simulink model "TST_FanSpd_DD"  (R2016b)
settings: Solver=FixedStepDiscrete  StartTime=0.0  StopTime=simTime  FixedStep=sampleTime  RelTol=1e-3
values from neighbouring files (symbols this model uses):
  testCase = 1    [initTST_FanSpd_DD_001.m]    (also in initTST_FanSpd_DD_002.m = 2)
libraries: simulink x7, UnitTest_Lib x4
settings Model: Creator=xinchangran  LastModifiedBy=xinchangran
settings DebuggingCC: SignalRangeChecking=error

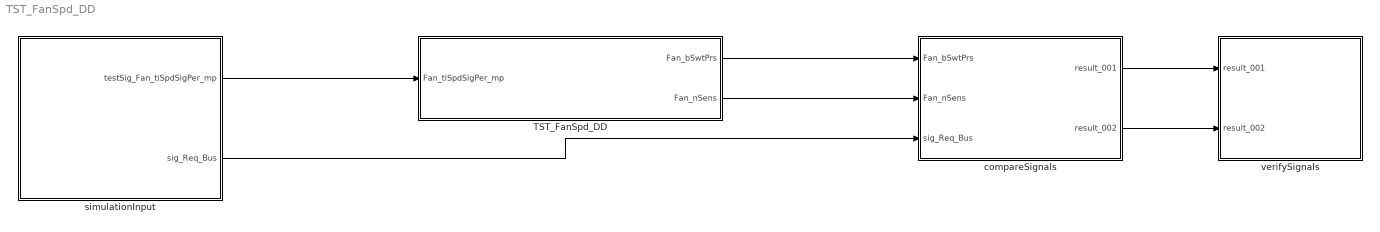
== system TST_FanSpd_DD ==
  TST_FanSpd_DD : Subsystem
  compareSignals : Subsystem
  simulationInput : Subsystem
  verifySignals : Subsystem
  wires:
  simulationInput/1(testSig_Fan_tiSpdSigPer_mp) -> TST_FanSpd_DD/1(Fan_tiSpdSigPer_mp)
  TST_FanSpd_DD/1(Fan_bSwtPrs) -> compareSignals/1(Fan_bSwtPrs)
  TST_FanSpd_DD/2(Fan_nSens) -> compareSignals/2(Fan_nSens)
  simulationInput/2(sig_Req_Bus) -> compareSignals/3(sig_Req_Bus)
  compareSignals/1(result_001) -> verifySignals/1(result_001)
  compareSignals/2(result_002) -> verifySignals/2(result_002)

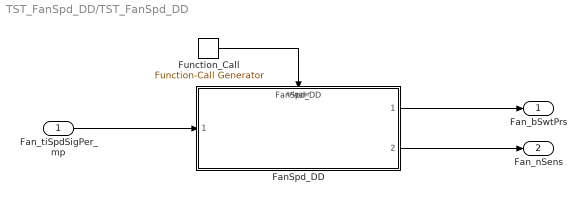
== system TST_FanSpd_DD/TST_FanSpd_DD ==
  Fan_tiSpdSigPer_mp : Inport
  FanSpd_DD : ModelReference  ModelNameDialog=FanSpd_DD  SimulationMode=Normal  ModelReferenceVersion=1.45  TriggerPortName=function  TriggerPortTriggerType=function-call  TriggerPortStatesWhenEnabling=held
  Function_Call : simulink/Ports & Subsystems/Function-Call Generator  sample_time=sampleTime  numberOfIterations=1
  Fan_bSwtPrs : Outport
  Fan_nSens : Outport  Port=2
  wires:
  Function_Call/1 -> FanSpd_DD/Trigger
  Fan_tiSpdSigPer_mp/1 -> FanSpd_DD/1
  FanSpd_DD/1 -> Fan_bSwtPrs/1
  FanSpd_DD/2 -> Fan_nSens/1

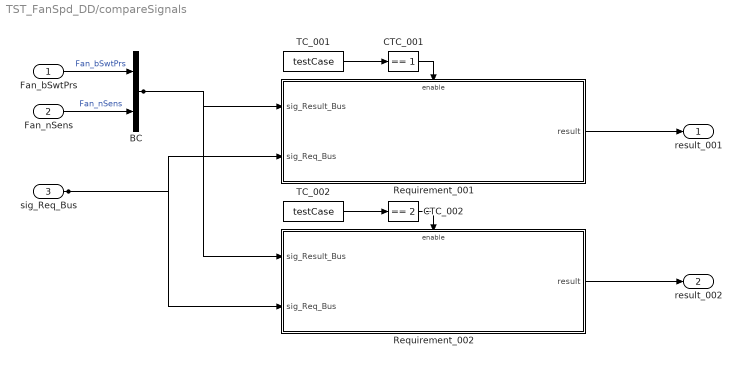
== system TST_FanSpd_DD/compareSignals ==
  Fan_bSwtPrs : Inport
  Fan_nSens : Inport  Port=2
  sig_Req_Bus : Inport  Port=3
  BC : BusCreator  Inputs=2
  CTC_001 : simulink/Logic and Bit Operations/Compare To Constant  relop===  const=1  OutDataTypeStr=boolean
  CTC_002 : simulink/Logic and Bit Operations/Compare To Constant  relop===  const=2  OutDataTypeStr=boolean
  Requirement_001 : Subsystem
  Requirement_002 : Subsystem
  TC_001 : Constant  Value=testCase
  TC_002 : Constant  Value=testCase
  result_001 : Outport
  result_002 : Outport  Port=2
  wires:
  Fan_bSwtPrs/1 -> BC/1  "Fan_bSwtPrs"
  Fan_nSens/1 -> BC/2  "Fan_nSens"
  TC_001/1 -> CTC_001/1
  CTC_001/1 -> Requirement_001/Enable
  sig_Req_Bus/1 -> Requirement_001/2(sig_Req_Bus), Requirement_002/2(sig_Req_Bus)
  BC/1 -> Requirement_001/1(sig_Result_Bus), Requirement_002/1(sig_Result_Bus)
  Requirement_001/1(result) -> result_001/1
  TC_002/1 -> CTC_002/1
  CTC_002/1 -> Requirement_002/Enable
  Requirement_002/1(result) -> result_002/1

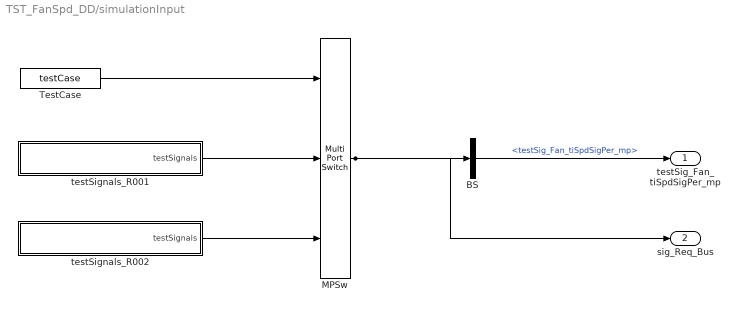
== system TST_FanSpd_DD/simulationInput ==
  BS : BusSelector  OutputSignals=testSig_Fan_tiSpdSigPer_mp
  MPSw : MultiPortSwitch  Inputs=2  SaturateOnIntegerOverflow=on  InputSameDT=on
  TestCase : Constant  Value=testCase
  testSignals_R001 : Subsystem
  testSignals_R002 : Subsystem
  testSig_Fan_tiSpdSigPer_mp : Outport
  sig_Req_Bus : Outport  Port=2
  wires:
  BS/1 -> testSig_Fan_tiSpdSigPer_mp/1  "<testSig_Fan_tiSpdSigPer_mp>"
  MPSw/1 -> BS/1, sig_Req_Bus/1
  TestCase/1 -> MPSw/1
  testSignals_R001/1(testSignals) -> MPSw/2
  testSignals_R002/1(testSignals) -> MPSw/3

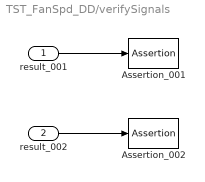
== system TST_FanSpd_DD/verifySignals ==
  result_001 : Inport
  result_002 : Inport  Port=2
  Assertion_001 : Assertion  Enabled=off
  Assertion_002 : Assertion  Enabled=off
  wires:
  result_001/1 -> Assertion_001/1
  result_002/1 -> Assertion_002/1

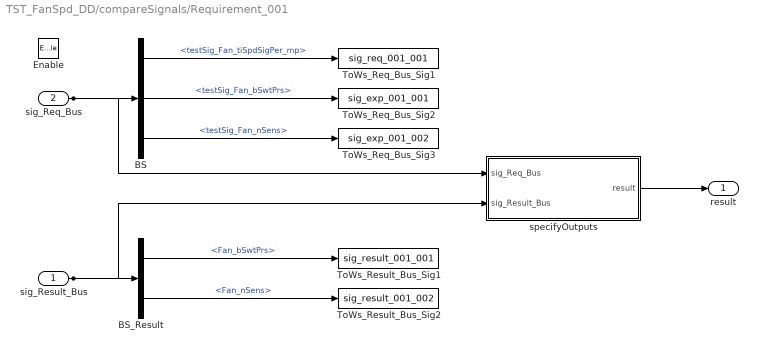
== system TST_FanSpd_DD/compareSignals/Requirement_001 ==
  sig_Result_Bus : Inport
  sig_Req_Bus : Inport  Port=2
  Enable : EnablePort
  BS : BusSelector  OutputSignals=testSig_Fan_tiSpdSigPer_mp,testSig_Fan_bSwtPrs,testSig_Fan_nSens
  BS_Result : BusSelector  OutputSignals=Fan_bSwtPrs,Fan_nSens
  ToWs_Req_Bus_Sig1 : ToWorkspace  VariableName=sig_req_001_001  SaveFormat=Structure With Time
  ToWs_Req_Bus_Sig2 : ToWorkspace  VariableName=sig_exp_001_001  SaveFormat=Structure With Time
  ToWs_Req_Bus_Sig3 : ToWorkspace  VariableName=sig_exp_001_002  SaveFormat=Structure With Time
  ToWs_Result_Bus_Sig1 : ToWorkspace  VariableName=sig_result_001_001  SaveFormat=Structure With Time
  ToWs_Result_Bus_Sig2 : ToWorkspace  VariableName=sig_result_001_002  SaveFormat=Structure With Time
  specifyOutputs : Subsystem
  result : Outport
  wires:
  sig_Req_Bus/1 -> BS/1, specifyOutputs/1(sig_Req_Bus)
  BS/1 -> ToWs_Req_Bus_Sig1/1  "<testSig_Fan_tiSpdSigPer_mp>"
  BS/2 -> ToWs_Req_Bus_Sig2/1  "<testSig_Fan_bSwtPrs>"
  BS/3 -> ToWs_Req_Bus_Sig3/1  "<testSig_Fan_nSens>"
  sig_Result_Bus/1 -> BS_Result/1, specifyOutputs/2(sig_Result_Bus)
  BS_Result/1 -> ToWs_Result_Bus_Sig1/1  "<Fan_bSwtPrs>"
  BS_Result/2 -> ToWs_Result_Bus_Sig2/1  "<Fan_nSens>"
  specifyOutputs/1(result) -> result/1

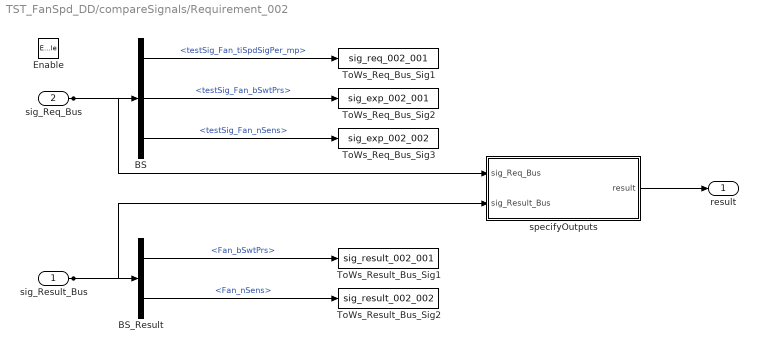
== system TST_FanSpd_DD/compareSignals/Requirement_002 ==
  sig_Result_Bus : Inport
  sig_Req_Bus : Inport  Port=2
  Enable : EnablePort
  BS : BusSelector  OutputSignals=testSig_Fan_tiSpdSigPer_mp,testSig_Fan_bSwtPrs,testSig_Fan_nSens
  BS_Result : BusSelector  OutputSignals=Fan_bSwtPrs,Fan_nSens
  ToWs_Req_Bus_Sig1 : ToWorkspace  VariableName=sig_req_002_001  SaveFormat=Structure With Time
  ToWs_Req_Bus_Sig2 : ToWorkspace  VariableName=sig_exp_002_001  SaveFormat=Structure With Time
  ToWs_Req_Bus_Sig3 : ToWorkspace  VariableName=sig_exp_002_002  SaveFormat=Structure With Time
  ToWs_Result_Bus_Sig1 : ToWorkspace  VariableName=sig_result_002_001  SaveFormat=Structure With Time
  ToWs_Result_Bus_Sig2 : ToWorkspace  VariableName=sig_result_002_002  SaveFormat=Structure With Time
  specifyOutputs : Subsystem
  result : Outport
  wires:
  sig_Req_Bus/1 -> BS/1, specifyOutputs/1(sig_Req_Bus)
  BS/1 -> ToWs_Req_Bus_Sig1/1  "<testSig_Fan_tiSpdSigPer_mp>"
  BS/2 -> ToWs_Req_Bus_Sig2/1  "<testSig_Fan_bSwtPrs>"
  BS/3 -> ToWs_Req_Bus_Sig3/1  "<testSig_Fan_nSens>"
  sig_Result_Bus/1 -> BS_Result/1, specifyOutputs/2(sig_Result_Bus)
  BS_Result/1 -> ToWs_Result_Bus_Sig1/1  "<Fan_bSwtPrs>"
  BS_Result/2 -> ToWs_Result_Bus_Sig2/1  "<Fan_nSens>"
  specifyOutputs/1(result) -> result/1

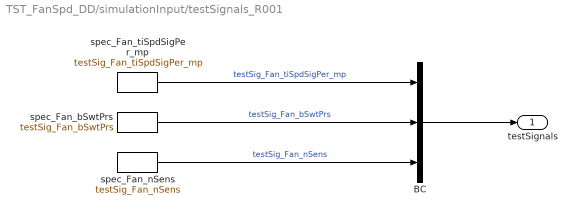
== system TST_FanSpd_DD/simulationInput/testSignals_R001 ==
  BC : BusCreator  Inputs=3
  spec_Fan_bSwtPrs : FromWorkspace  VariableName=testSig_Fan_bSwtPrs  Interpolate=off  OutputAfterFinalValue=Holding final value
  spec_Fan_nSens : FromWorkspace  VariableName=testSig_Fan_nSens  Interpolate=off  OutputAfterFinalValue=Holding final value
  spec_Fan_tiSpdSigPer_mp : FromWorkspace  VariableName=testSig_Fan_tiSpdSigPer_mp  Interpolate=off  OutputAfterFinalValue=Holding final value
  testSignals : Outport
  wires:
  BC/1 -> testSignals/1
  spec_Fan_tiSpdSigPer_mp/1 -> BC/1  "testSig_Fan_tiSpdSigPer_mp"
  spec_Fan_bSwtPrs/1 -> BC/2  "testSig_Fan_bSwtPrs"
  spec_Fan_nSens/1 -> BC/3  "testSig_Fan_nSens"

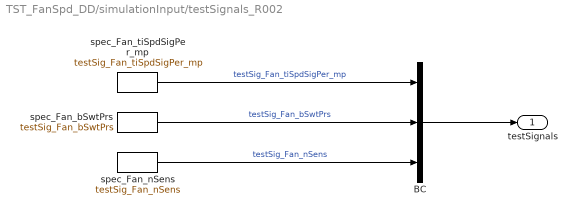
== system TST_FanSpd_DD/simulationInput/testSignals_R002 ==
  BC : BusCreator  Inputs=3
  spec_Fan_bSwtPrs : FromWorkspace  VariableName=testSig_Fan_bSwtPrs  Interpolate=off  OutputAfterFinalValue=Holding final value
  spec_Fan_nSens : FromWorkspace  VariableName=testSig_Fan_nSens  Interpolate=off  OutputAfterFinalValue=Holding final value
  spec_Fan_tiSpdSigPer_mp : FromWorkspace  VariableName=testSig_Fan_tiSpdSigPer_mp  Interpolate=off  OutputAfterFinalValue=Holding final value
  testSignals : Outport
  wires:
  BC/1 -> testSignals/1
  spec_Fan_tiSpdSigPer_mp/1 -> BC/1  "testSig_Fan_tiSpdSigPer_mp"
  spec_Fan_bSwtPrs/1 -> BC/2  "testSig_Fan_bSwtPrs"
  spec_Fan_nSens/1 -> BC/3  "testSig_Fan_nSens"

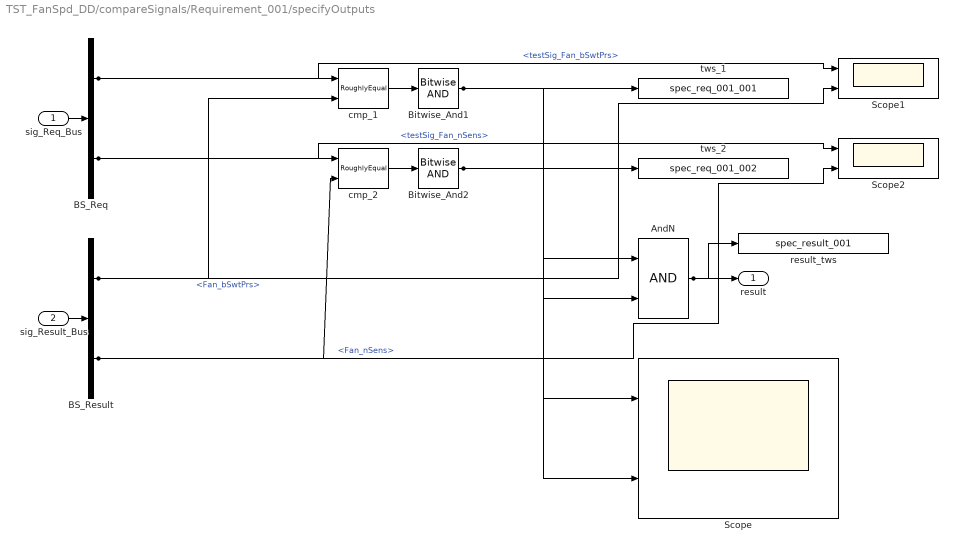
== system TST_FanSpd_DD/compareSignals/Requirement_001/specifyOutputs ==
  sig_Req_Bus : Inport
  sig_Result_Bus : Inport  Port=2
  AndN : Logic
  BS_Req : BusSelector  OutputSignals=testSig_Fan_bSwtPrs,testSig_Fan_nSens
  BS_Result : BusSelector  OutputSignals=Fan_bSwtPrs,Fan_nSens
  Bitwise_And1 : simulink/Logic and Bit Operations/Bitwise Operator  logicop=AND  UseBitMask=off  BitMask=bin2dec('11011001')  BitMaskRealWorld=Stored Integer
  Bitwise_And2 : simulink/Logic and Bit Operations/Bitwise Operator  logicop=AND  UseBitMask=off  BitMask=bin2dec('11011001')  BitMaskRealWorld=Stored Integer
  Scope : Scope  NumInputPorts=2
  Scope1 : Scope  NumInputPorts=2
  Scope2 : Scope  NumInputPorts=2
  cmp_1 : UnitTest_Lib/RoughlyEqual  slope=0.1
  cmp_2 : UnitTest_Lib/RoughlyEqual  slope=0.1
  result_tws : ToWorkspace  VariableName=spec_result_001
  tws_1 : ToWorkspace  VariableName=spec_req_001_001
  tws_2 : ToWorkspace  VariableName=spec_req_001_002
  result : Outport
  wires:
  sig_Req_Bus/1 -> BS_Req/1
  sig_Result_Bus/1 -> BS_Result/1
  AndN/1 -> result/1, result_tws/1
  BS_Req/1 -> cmp_1/1, Scope1/1  "<testSig_Fan_bSwtPrs>"
  BS_Result/1 -> cmp_1/2, Scope1/2  "<Fan_bSwtPrs>"
  cmp_1/1 -> Bitwise_And1/1
  Bitwise_And1/1 -> tws_1/1, AndN/1, Scope/1
  BS_Req/2 -> cmp_2/1, Scope2/1  "<testSig_Fan_nSens>"
  BS_Result/2 -> cmp_2/2, Scope2/2  "<Fan_nSens>"
  cmp_2/1 -> Bitwise_And2/1
  Bitwise_And2/1 -> tws_2/1, AndN/2, Scope/2

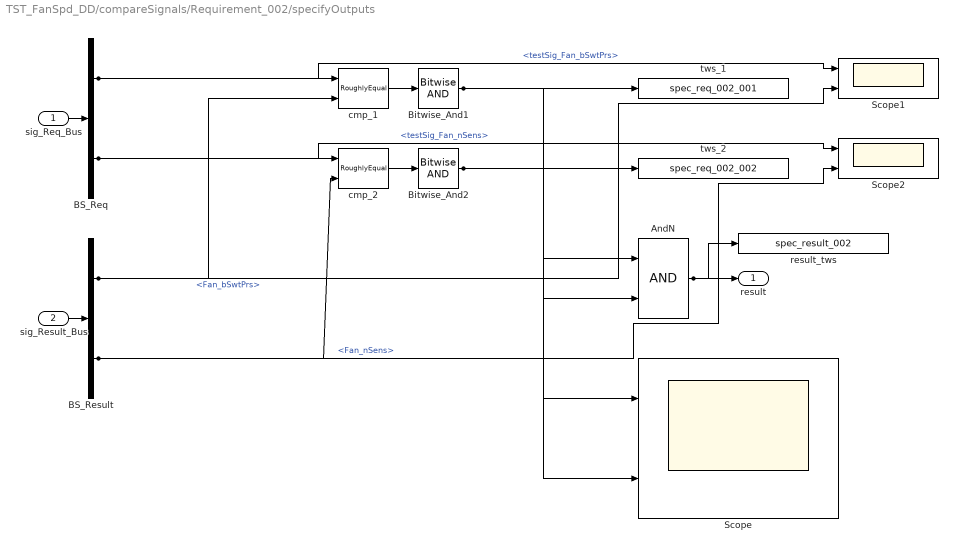
== system TST_FanSpd_DD/compareSignals/Requirement_002/specifyOutputs ==
  sig_Req_Bus : Inport
  sig_Result_Bus : Inport  Port=2
  AndN : Logic
  BS_Req : BusSelector  OutputSignals=testSig_Fan_bSwtPrs,testSig_Fan_nSens
  BS_Result : BusSelector  OutputSignals=Fan_bSwtPrs,Fan_nSens
  Bitwise_And1 : simulink/Logic and Bit Operations/Bitwise Operator  logicop=AND  UseBitMask=off  BitMask=bin2dec('11011001')  BitMaskRealWorld=Stored Integer
  Bitwise_And2 : simulink/Logic and Bit Operations/Bitwise Operator  logicop=AND  UseBitMask=off  BitMask=bin2dec('11011001')  BitMaskRealWorld=Stored Integer
  Scope : Scope  NumInputPorts=2
  Scope1 : Scope  NumInputPorts=2
  Scope2 : Scope  NumInputPorts=2
  cmp_1 : UnitTest_Lib/RoughlyEqual  slope=0.1
  cmp_2 : UnitTest_Lib/RoughlyEqual  slope=0.1
  result_tws : ToWorkspace  VariableName=spec_result_002
  tws_1 : ToWorkspace  VariableName=spec_req_002_001
  tws_2 : ToWorkspace  VariableName=spec_req_002_002
  result : Outport
  wires:
  sig_Req_Bus/1 -> BS_Req/1
  sig_Result_Bus/1 -> BS_Result/1
  AndN/1 -> result/1, result_tws/1
  BS_Req/1 -> cmp_1/1, Scope1/1  "<testSig_Fan_bSwtPrs>"
  BS_Result/1 -> cmp_1/2, Scope1/2  "<Fan_bSwtPrs>"
  cmp_1/1 -> Bitwise_And1/1
  Bitwise_And1/1 -> tws_1/1, AndN/1, Scope/1
  BS_Req/2 -> cmp_2/1, Scope2/1  "<testSig_Fan_nSens>"
  BS_Result/2 -> cmp_2/2, Scope2/2  "<Fan_nSens>"
  cmp_2/1 -> Bitwise_And2/1
  Bitwise_And2/1 -> tws_2/1, AndN/2, Scope/2
